simulink model "menablesubsys"  (Simulink 8.0)
settings: Solver=FixedStepDiscrete  StartTime=0.0  StopTime=10.0  FixedStep=1  RelTol=1e-3
settings Model: Creator=mtocci  LastModifiedBy=mtocci
settings DataIOCC: LimitDataPoints=off  SaveFormat=StructureWithTime  SignalLoggingSaveFormat=ModelDataLogs
settings OptimizationCC: InlineParams=on
settings DebuggingCC: FcnCallInpInsideContextMsg=Use local settings  StrictBusMsg=ErrorOnBusTreatedAsVector
settings GRTTargetCC: CombineOutputUpdateFcns=off

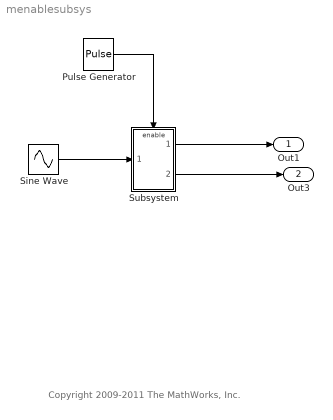
== system menablesubsys ==
  note: Copyright 2009-2011 The MathWorks, Inc.
  Pulse Generator : DiscretePulseGenerator  Amplitude=[1 1 2 2]
  Sine Wave : Sin  SineType=Sample based  Samples=5  SampleTime=1
  Subsystem : Subsystem
  Out1 : Outport  InitialOutput=0
  Out3 : Outport  Port=2  InitialOutput=0
  wires:
  Subsystem/1(Out1) -> Out1/1
  Subsystem/2(Out3) -> Out3/1
  Sine Wave/1 -> Subsystem/1(In2)
  Pulse Generator/1 -> Subsystem/Enable

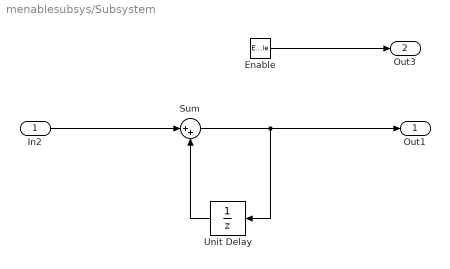
== system menablesubsys/Subsystem ==
  In2 : Inport
  Enable : EnablePort  ShowOutputPort=on
  Sum : Sum  Inputs=|++
  Unit Delay : UnitDelay  SampleTime=-1
  Out1 : Outport  InitialOutput=0
  Out3 : Outport  Port=2  InitialOutput=0
  wires:
  In2/1 -> Sum/1
  Sum/1 -> Out1/1, Unit Delay/1
  Unit Delay/1 -> Sum/2
  Enable/1 -> Out3/1
